simulink subsystem "Environment"  (R2019b)
settings: Solver=VariableStepAuto  StartTime=0.0  StopTime=10.0  RelTol=1e-3
undefined symbols (not defined in the file): base_windspeed, ENVMT
libraries: simulink_extras x1
settings Model: Creator=dylaneijkelhof  LastModifiedBy=dylaneijkelhof

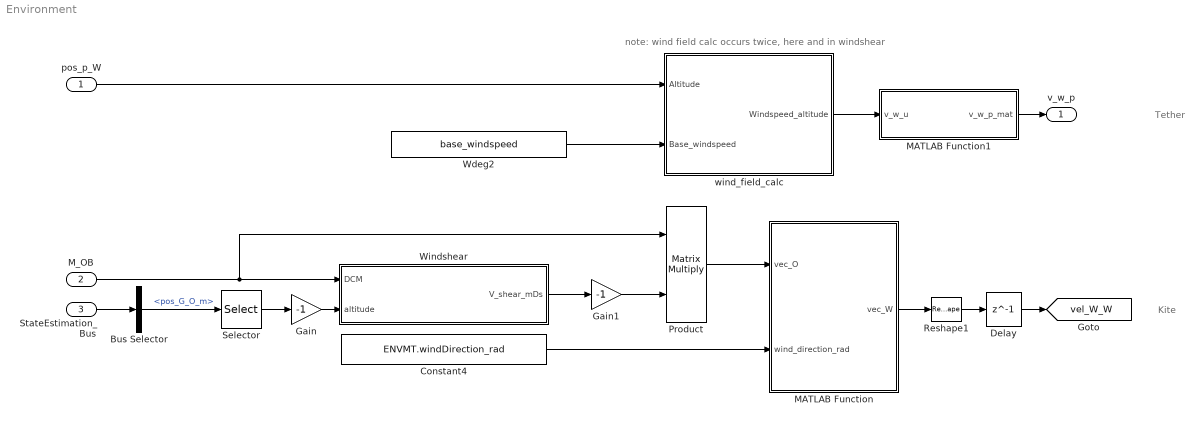
== system Environment ==
  note: note: wind field calc occurs twice, here and in windshear
  note: Kite
  note: Tether
  pos_p_W : Inport
  M_OB : Inport  Port=2
  StateEstimation_Bus : Inport  Port=3
  Bus Selector : BusSelector  OutputSignals=pos_G_O_m
  Constant4 : Constant  Value=ENVMT.windDirection_rad
  Delay : Delay  DelayLength=1  InitialCondition=zeros(3,1)
  Gain : Gain  Gain=-1
  Gain1 : Gain  Gain=-1
  MATLAB Function : MATLAB Function  TreatAsAtomicUnit=on
  MATLAB Function1 : MATLAB Function  TreatAsAtomicUnit=on
  Product : Product  Multiplication=Matrix(*)
  Reshape1 : Reshape  OutputDimensionality=Column vector (2-D)
  Selector : Selector  InputPortWidth=3  IndexOptions=Index vector (dialog)  Indices=3  OutputSizes=1
  Wdeg2 : Constant  Value=base_windspeed  OutDataTypeStr=Inherit: Inherit via back propagation
  Windshear : Subsystem
  wind_field_calc : Subsystem
  v_w_p : Outport  VectorParamsAs1DForOutWhenUnconnected=off
  tag scope: vel_W_W=global
  wires:
  Bus Selector/1 -> Selector/1  "<pos_G_O_m>"
  Selector/1 -> Gain/1
  MATLAB Function/1(vec_W) -> Reshape1/1
  StateEstimation_Bus/1 -> Bus Selector/1
  Product/1 -> MATLAB Function/1(vec_O)
  M_OB/1 -> Product/1, Windshear/1(DCM)
  Windshear/1(V_shear_mDs) -> Gain1/1
  Gain1/1 -> Product/2
  Gain/1 -> Windshear/2(altitude)
  Constant4/1 -> MATLAB Function/2(wind_direction_rad)
  Reshape1/1 -> Delay/1
  pos_p_W/1 -> wind_field_calc/1(Altitude)
  MATLAB Function1/1(v_w_p_mat) -> v_w_p/1
  Delay/1 -> [vel_W_W]
  Wdeg2/1 -> wind_field_calc/2(Base_windspeed)
  wind_field_calc/1(Windspeed_altitude) -> MATLAB Function1/1(v_w_u)

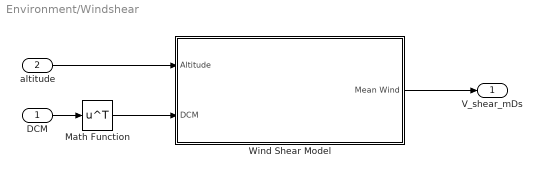
== system Environment/Windshear ==
  DCM : Inport
  altitude : Inport  Port=2
  Math Function : Math  Operator=transpose  SaturateOnIntegerOverflow=on
  Wind Shear Model : Subsystem
  V_shear_mDs : Outport  VectorParamsAs1DForOutWhenUnconnected=off
  wires:
  Wind Shear Model/1(Mean Wind) -> V_shear_mDs/1
  Math Function/1 -> Wind Shear Model/2(DCM)
  DCM/1 -> Math Function/1
  altitude/1 -> Wind Shear Model/1(Altitude)

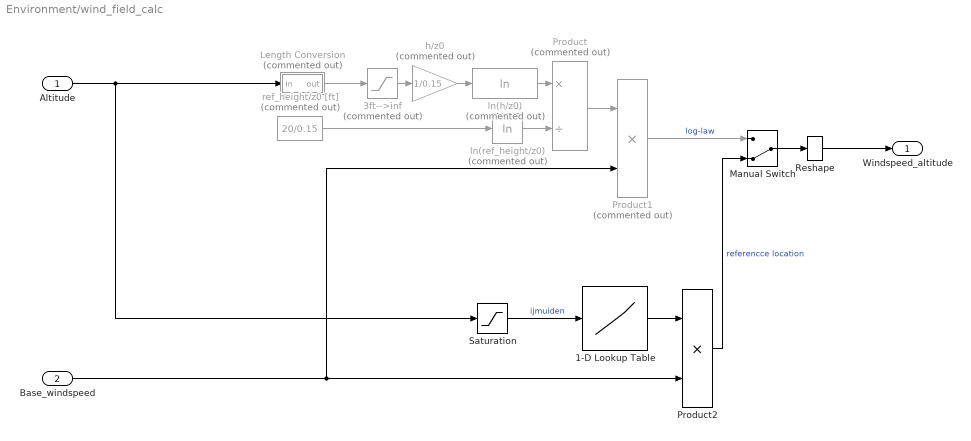
== system Environment/wind_field_calc ==
  Altitude : Inport
  Base_windspeed : Inport  Port=2
  1-D Lookup Table : Lookup_n-D  NumberOfTableDimensions=1  BreakpointsForDimension1=ENVMT.wind_height  Table=ENVMT.wind_data  InternalRulePriority=Speed  RndMeth=Simplest  InputSameDT=on
  3ft-->inf : Saturate  Commented=on  UpperLimit=inf  LowerLimit=3
  Length Conversion : Subsystem  Commented=on
  Manual Switch : ManualSwitch  CurrentSetting=0
  Product : Product  Commented=on  Inputs=*/  SaturateOnIntegerOverflow=on  InputSameDT=on  OutDataTypeStr=Inherit: Same as first input
  Product1 : Product  Commented=on  SaturateOnIntegerOverflow=on  InputSameDT=on  OutDataTypeStr=Inherit: Same as first input
  Product2 : Product  SaturateOnIntegerOverflow=on  InputSameDT=on  OutDataTypeStr=Inherit: Same as first input
  Reshape : Reshape  OutputDimensionality=Column vector (2-D)
  Saturation : Saturate  UpperLimit=ENVMT.height_max  LowerLimit=ENVMT.wind_height(1)
  h/z0 : Gain  Commented=on  Gain=1/0.15  SaturateOnIntegerOverflow=on  OutDataTypeStr=Inherit: Same as input  ParamDataTypeStr=Inherit: Same as input
  ln(h/z0) : Math  Commented=on  Operator=log  SaturateOnIntegerOverflow=on
  ln(ref_height/z0) : Math  Commented=on  Operator=log  SaturateOnIntegerOverflow=on
  ref_height/z0 [ft] : Constant  Commented=on  Value=20/0.15  OutDataTypeStr=Inherit: Inherit via back propagation
  Windspeed_altitude : Outport
  wires:
  3ft-->inf/1 -> h/z0/1
  Product2/1 -> Manual Switch/2  "referencce location"
  ln(ref_height/z0)/1 -> Product/2
  1-D Lookup Table/1 -> Product2/1
  Reshape/1 -> Windspeed_altitude/1
  ln(h/z0)/1 -> Product/1
  Length Conversion/1(out) -> 3ft-->inf/1
  Product1/1 -> Manual Switch/1  "log-law"
  Base_windspeed/1 -> Product1/2, Product2/2
  Saturation/1 -> 1-D Lookup Table/1  "ijmuiden"
  Manual Switch/1 -> Reshape/1
  Product/1 -> Product1/1
  h/z0/1 -> ln(h/z0)/1
  ref_height/z0 [ft]/1 -> ln(ref_height/z0)/1
  Altitude/1 -> Length Conversion/1(in), Saturation/1

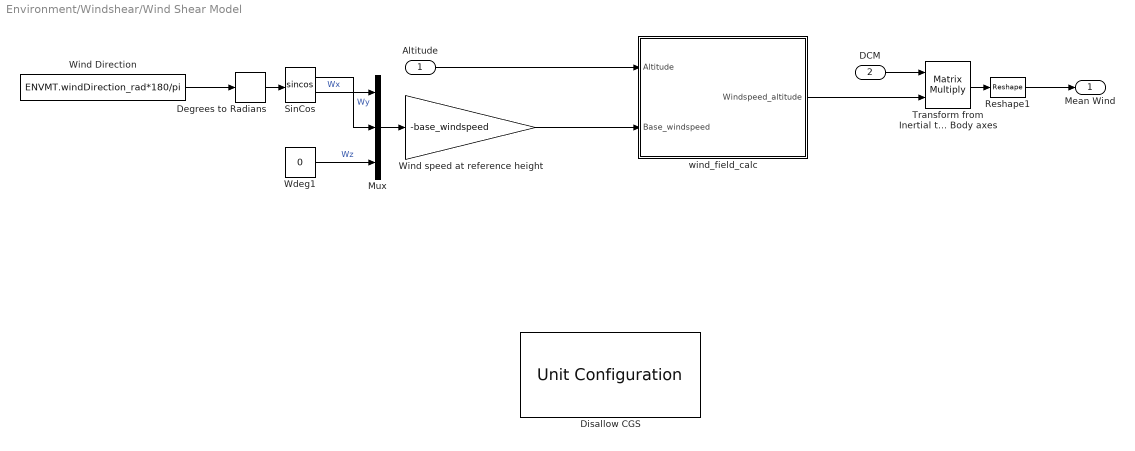
== system Environment/Windshear/Wind Shear Model ==
  Altitude : Inport  Unit=m
  DCM : Inport  Port=2  Unit=1  PortDimensions=[3 3]
  Degrees to Radians : simulink_extras/Transformations/Degrees to Radians
  Disallow CGS : UnitConfiguration  UnitSystemsStr=English,SI,SI (extended)  AllowAllUnitSystems=off
  Mux : Mux  Inputs=3
  Reshape1 : Reshape
  SinCos : Trigonometry  Operator=sincos
  Transform from Inertial to Body axes : Product  Inputs=**  Multiplication=Matrix(*)  SaturateOnIntegerOverflow=on  InputSameDT=on  OutDataTypeStr=Inherit: Same as first input
  Wdeg1 : Constant  Value=0  OutDataTypeStr=Inherit: Inherit via back propagation
  Wind Direction : Constant  Value=ENVMT.windDirection_rad*180/pi  OutDataTypeStr=Inherit: Inherit via back propagation
  Wind speed at reference height : Gain  Gain=-base_windspeed  SaturateOnIntegerOverflow=on  OutDataTypeStr=Inherit: Same as input  ParamDataTypeStr=Inherit: Same as input
  wind_field_calc : Subsystem
  Mean Wind : Outport  Unit=m/s  VectorParamsAs1DForOutWhenUnconnected=off
  wires:
  Altitude/1 -> wind_field_calc/1(Altitude)
  Transform from Inertial to Body axes/1 -> Reshape1/1
  Wind Direction/1 -> Degrees to Radians/1
  SinCos/2 -> Mux/1  "Wx"
  SinCos/1 -> Mux/2  "Wy"
  Wdeg1/1 -> Mux/3  "Wz"
  Mux/1 -> Wind speed at reference height/1
  DCM/1 -> Transform from Inertial to Body axes/1
  Wind speed at reference height/1 -> wind_field_calc/2(Base_windspeed)
  Degrees to Radians/1 -> SinCos/1
  wind_field_calc/1(Windspeed_altitude) -> Transform from Inertial to Body axes/2
  Reshape1/1 -> Mean Wind/1

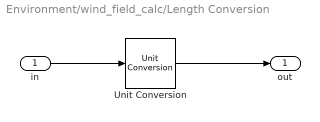
== system Environment/wind_field_calc/Length Conversion ==
  in : Inport  Unit=m
  Unit Conversion : UnitConversion
  out : Outport  Unit=ft  VectorParamsAs1DForOutWhenUnconnected=off
  wires:
  in/1 -> Unit Conversion/1
  Unit Conversion/1 -> out/1

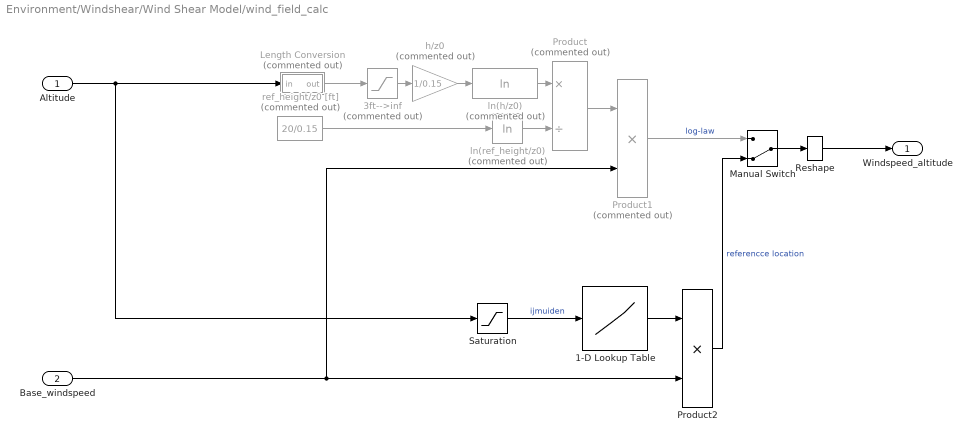
== system Environment/Windshear/Wind Shear Model/wind_field_calc ==
  Altitude : Inport
  Base_windspeed : Inport  Port=2
  1-D Lookup Table : Lookup_n-D  NumberOfTableDimensions=1  BreakpointsForDimension1=ENVMT.wind_height  Table=ENVMT.wind_data  InternalRulePriority=Speed  RndMeth=Simplest  InputSameDT=on
  3ft-->inf : Saturate  Commented=on  UpperLimit=inf  LowerLimit=3
  Length Conversion : Subsystem  Commented=on
  Manual Switch : ManualSwitch  CurrentSetting=0
  Product : Product  Commented=on  Inputs=*/  SaturateOnIntegerOverflow=on  InputSameDT=on  OutDataTypeStr=Inherit: Same as first input
  Product1 : Product  Commented=on  SaturateOnIntegerOverflow=on  InputSameDT=on  OutDataTypeStr=Inherit: Same as first input
  Product2 : Product  SaturateOnIntegerOverflow=on  InputSameDT=on  OutDataTypeStr=Inherit: Same as first input
  Reshape : Reshape  OutputDimensionality=Column vector (2-D)
  Saturation : Saturate  UpperLimit=ENVMT.height_max  LowerLimit=ENVMT.wind_height(1)
  h/z0 : Gain  Commented=on  Gain=1/0.15  SaturateOnIntegerOverflow=on  OutDataTypeStr=Inherit: Same as input  ParamDataTypeStr=Inherit: Same as input
  ln(h/z0) : Math  Commented=on  Operator=log  SaturateOnIntegerOverflow=on
  ln(ref_height/z0) : Math  Commented=on  Operator=log  SaturateOnIntegerOverflow=on
  ref_height/z0 [ft] : Constant  Commented=on  Value=20/0.15  OutDataTypeStr=Inherit: Inherit via back propagation
  Windspeed_altitude : Outport
  wires:
  3ft-->inf/1 -> h/z0/1
  Product2/1 -> Manual Switch/2  "referencce location"
  ln(ref_height/z0)/1 -> Product/2
  1-D Lookup Table/1 -> Product2/1
  Reshape/1 -> Windspeed_altitude/1
  ln(h/z0)/1 -> Product/1
  Length Conversion/1(out) -> 3ft-->inf/1
  Product1/1 -> Manual Switch/1  "log-law"
  Base_windspeed/1 -> Product1/2, Product2/2
  Saturation/1 -> 1-D Lookup Table/1  "ijmuiden"
  Manual Switch/1 -> Reshape/1
  Product/1 -> Product1/1
  h/z0/1 -> ln(h/z0)/1
  ref_height/z0 [ft]/1 -> ln(ref_height/z0)/1
  Altitude/1 -> Length Conversion/1(in), Saturation/1

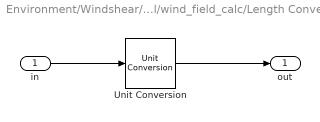
== system Environment/Windshear/Wind Shear Model/wind_field_calc/Length Conversion ==
  in : Inport  Unit=m
  Unit Conversion : UnitConversion
  out : Outport  Unit=ft  VectorParamsAs1DForOutWhenUnconnected=off
  wires:
  in/1 -> Unit Conversion/1
  Unit Conversion/1 -> out/1

== matlab function Environment/MATLAB Function ==
  data: vec_W output; vec_O input; wind_direction_rad input
% Copyright 2021 Delft University of Technology
%
% Licensed under the Apache License, Version 2.0 (the "License");
% you may not use this file except in compliance with the License.
% You may obtain a copy of the License at
%
%      http://www.apache.org/licenses/LICENSE-2.0
%
% Unless required by applicable law or agreed to in writing, software
% distributed under the License is distributed on an "AS IS" BASIS,
% WITHOUT WARRANTIES OR CONDITIONS OF ANY KIND, either express or implied.
% See the License for the specific language governing permissions and
% limitations under the License.

function vec_W = transformO2W(vec_O, wind_direction_rad)
%transformO2W - transform inertial reference frame to wind reference frame
%
% Syntax:  vec_W = transformO2W(vec_O, wind_direction_rad)
%
% Inputs:
%    vec_O - Aircraft position in inertial reference frame
%    wind_direction_rad - Wind direction angle compared to intertial
%                         reference frame
%
% Outputs:
%    vec_W  - Propulsive forces in body reference frame
%   
% Example: 
%    vec_W = transformO2W(vec_O, wind_direction_rad)
%
% Other m-files required: none
% Subfunctions: none
% MAT-files required: none
%
% Author: Dylan Eijkelhof, M.Sc.
% Delft University of Technology
% email address: d.eijkelhof@tudelft.nl  
% December 2019; Last revision: 30-September-2019

%------------- BEGIN CODE --------------    

M_WO = [cos(wind_direction_rad), sin(wind_direction_rad), 0;
        sin(wind_direction_rad), -cos(wind_direction_rad), 0;
        0, 0, -1];

vec_W = M_WO*vec_O;
%------------- END CODE --------------   
end

== matlab function Environment/MATLAB Function1 ==
  data: v_w_u input; v_w_p_mat output
% Copyright 2021 Delft University of Technology
%
% Licensed under the Apache License, Version 2.0 (the "License");
% you may not use this file except in compliance with the License.
% You may obtain a copy of the License at
%
%      http://www.apache.org/licenses/LICENSE-2.0
%
% Unless required by applicable law or agreed to in writing, software
% distributed under the License is distributed on an "AS IS" BASIS,
% WITHOUT WARRANTIES OR CONDITIONS OF ANY KIND, either express or implied.
% See the License for the specific language governing permissions and
% limitations under the License.

function v_w_p_mat = fcn(v_w_u)

v_w_p_mat = zeros( 3, length( v_w_u) );
v_w_p_mat(1,:) = v_w_u';
